simulink model "soc_estimation"  (R2024b)
settings: Solver=FixedStepAuto  StartTime=0.0  StopTime=6*3600  RelTol=1e-3
undefined symbols (not defined in the file): R, Ts
libraries: BatteryEstimators x8, simulink x4, nesl_utility x4, fl_lib x3, batteryecm_lib x1
settings Model: Creator=andri  LastModifiedBy=andri
settings OptimizationCC: DefaultParameterBehavior=Inlined  UseDivisionForNetSlopeComputation=on  GainParamInheritBuiltInType=on  UseFloatMulNetSlope=on  InlineInvariantSignals=on  EnhancedBackFolding=on  PassReuseOutputArgsAs=Individual arguments  ZeroExternalMemoryAtStartup=off  ZeroInternalMemoryAtStartup=off  EfficientFloat2IntCast=on  OptimizeBlockOrder=speed  DifferentSizesBufferReuse=on  OptimizationCustomize=off  EfficientTunableParamExpr=on
settings DebuggingCC: ParameterTunabilityLossMsg=error  SFUnexpectedBacktrackingDiag=warning  SFNoUnconditionalDefaultTransitionDiag=warning
settings HardwareCC: TargetBitPerLong=64  TargetBitPerPointer=64  TargetBitPerSizeT=64  TargetBitPerPtrDiffT=64  TargetLongLongMode=on  TargetIntDivRoundTo=Zero  TargetEndianess=LittleEndian  TargetWordSize=64  TargetHWDeviceType=MATLAB Host  ProdEqTarget=off
settings SFSimCC: MATLABDynamicMemAlloc=off  SimTargetLang=C++
settings RTWCC: Description=AUTOSAR  SystemTargetFile=autosar.tlc  GenCodeOnly=on  TemplateMakefile=ert_default_tmf  GenerateReport=on  BuildConfiguration=Debug  LaunchReport=on  DataTypeReplacement=CDataTypesFixedWidth
settings CodeAppCC: ForceParamTrailComments=on  IgnoreCustomStorageClasses=off  OperatorAnnotations=on  SimulinkDataObjDesc=on  SFDataObjDesc=on  InsertBlockDesc=on  EnableCustomComments=on
settings STFCustomTargetCC: TargetLangStandard=C99 (ISO)  MultiwordLength=256  ParMdlRefBuildCompliant=on  CompOptLevelCompliant=on  IncludeMdlTerminateFcn=off  CombineOutputUpdateFcns=on  SuppressErrorStatus=on  ERTCustomFileBanners=on  SupportNonFinite=off  SupportComplex=off  SupportContinuousTime=off  SupportNonInlinedSFcns=off  RemoveResetFunc=on  MATLABClassNameForMDSCustomization=Simulink.SoftwareTarget.ERTCustomization  AutosarCompliant=on  UseToolchainInfoCompliant=on  LookupTableObjectStructAxisOrder=2,1,3,4,...  LUTObjectStructOrderEvenSpacing=Size,Table,Breakpoints  SystemTargetFile=autosar.tlc
settings ERTTargetCC: TargetLangStandard=C99 (ISO)  ConcurrentExecutionCompliant=off  IncludeMdlTerminateFcn=off  SuppressErrorStatus=on  SupportNonFinite=off  SupportComplex=off  ModelStepFunctionPrototypeControlCompliant=off  CPPClassGenCompliant=off  AutosarCompliant=on  LookupTableObjectStructAxisOrder=2,1,3,4,...  LUTObjectStructOrderEvenSpacing=Size,Table,Breakpoints  ERTCustomFileTemplate=example_file_process.tlc  BooleanTrueId=TRUE  BooleanFalseId=FALSE

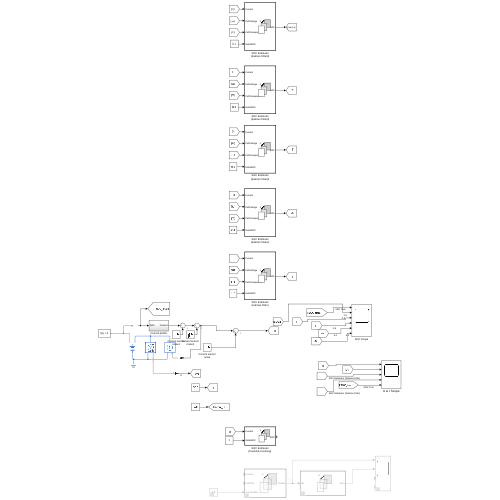
[thumbnail: Simulink's stored preview of the top-level diagram]
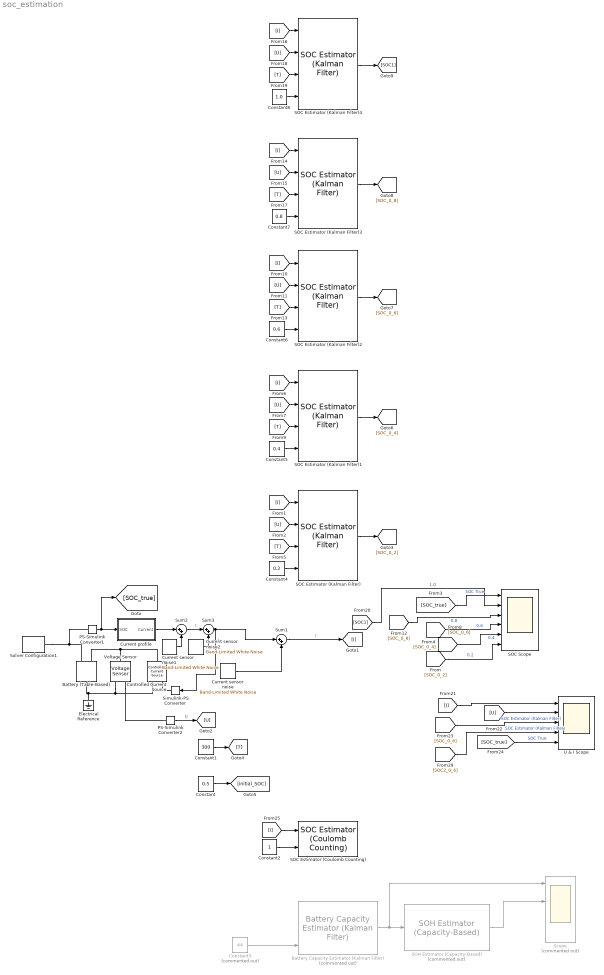
== system soc_estimation ==
  Battery (Table-Based) : batteryecm_lib/Battery (Table-Based)  SOC_vec=SOC  T_dependence=simscape.enum.tablebattery.temperature_dependence.yes  prm_dir=simscape.enum.tablebattery.prm_dir.noCurrentDirectionality  T_vec=T K  V0_mat=Em V  V0_vec=[3.5057, 3.566, 3.6337, 3.7127, 3.9259, 4.0777, 4.1928] V  V_range=[0, inf] V  R0_mat=R0 Ohm  R0_vec=[.0085, .0085, .0087, .0082, .0083, .0085, .0085] Ohm  R0_dis_mat=[.0117, .0085, .009; .011, .0085, .009; .0114, .0087, .0092; .0107, .0082, .0088; .0107, .0083, .0091; .0113, .0085, .0089; .0116, .0085, .0089] Ohm  R0_dis_vec=[.0085, .0085, .0087, .0082, .0083, .0085, .0085] Ohm  R0_ch_mat=[.0117, .0085, .009; .011, .0085, .009; .0114, .0087, .0092; .0107, .0082, .0088; .0107, .0083, .0091; .0113, .0085, .0089; .0116, .0085, .0089] Ohm  R0_ch_vec=[.0085, .0085, .0087, .0082, .0083, .0085, .0085] Ohm  AH=44 A*hr  prm_leak=simscape.enum.tablebattery.prm_leak.disabled  Rleak_vec=[8000, 7000, 6000] Ohm  Rleak=7e3 Ohm  extrapolation_option=simscape.enum.extrapolation.linear  SOC_port=simscape.enum.tablebattery.enable.yes  prm_dyn=simscape.enum.tablebattery.prm_dyn.rc2  R1_mat=R1 Ohm  R1_vec=[.0029, .0024, .0026, .0016, .0023, .0018, .0017] Ohm  tau1_mat=T1 s  tau1_vec=[36, 45, 105, 29, 77, 33, 39] s  R2_mat=R2 Ohm  R2_vec=[.0029, .0024, .0026, .0016, .0023, .0018, .0017] Ohm  tau2_mat=T2 s  tau2_vec=[36, 45, 105, 29, 77, 33, 39] s  R3_mat=[.0109, .0029, .0013; .0069, .0024, .0012; .0047, .0026, .0013; .0034, .0016, .001; .0033, .0023, .0014; .0033, .0018, .0011; .0028, .0017, .0011] Ohm  R3_vec=[.0029, .0024, .0026, .0016, .0023, .0018, .0017] Ohm  tau3_mat=[20, 36, 39; 31, 45, 39; 109, 105, 61; 36, 29, 26; 59, 77, 67; 40, 33, 29; 25, 39, 33] s  tau3_vec=[36, 45, 105, 29, 77, 33, 39] s  R4_mat=[.0109, .0029, .0013; .0069, .0024, .0012; .0047, .0026, .0013; .0034, .0016, .001; .0033, .0023, .0014; .0033, .0018, .0011; .0028, .0017, .0011] Ohm  R4_vec=[.0029, .0024, .0026, .0016, .0023, .0018, .0017] Ohm  tau4_mat=[20, 36, 39; 31, 45, 39; 109, 105, 61; 36, 29, 26; 59, 77, 67; 40, 33, 29; 25, 39, 33] s  tau4_vec=[36, 45, 105, 29, 77, 33, 39] s  R5_mat=[.0109, .0029, .0013; .0069, .0024, .0012; .0047, .0026, .0013; .0034, .0016, .001; .0033, .0023, .0014; .0033, .0018, .0011; .0028, .0017, .0011] Ohm  R5_vec=[.0029, .0024, .0026, .0016, .0023, .0018, .0017] Ohm  tau5_mat=[20, 36, 39; 31, 45, 39; 109, 105, 61; 36, 29, 26; 59, 77, 67; 40, 33, 29; 25, 39, 33] s  tau5_vec=[36, 45, 105, 29, 77, 33, 39] s  prm_fade=simscape.enum.tablebattery.prm_fade.tableN  N0=100  dV0=0  dR0=0  dAH=0  dRleak=0  dR1=0  dR2=0  dR3=0  dR4=0  dR5=0  N0vec=[1,5,10,20,30]  Tfadevec=[298.15, 323.15] K  dV0vec=[0, 0, 0, 0, 0]  dR0vec=[0, 0, 0, 0, 0]  dAHvec=[-1.0, 2.5, -5.0, -7.5, -10.0]  dRleakvec=[0, 0, 0, 0]  dR1vec=[0, 0, 0, 0, 0]  dR2vec=[0, 0, 0, 0, 0]  dR3vec=[0, 0, 0, 0]  dR4vec=[0, 0, 0, 0]  dR5vec=[0, 0, 0, 0]  dV0mat=[0, 0; 0, 0; 0, 0; 0, 0]  dR0mat=[0, 0; 0, 0; 0, 0; 0, 0]  dAHmat=[0, 0; 0, 0; 0, 0; 0, 0]  dRleakmat=[0, 0; 0, 0; 0, 0; 0, 0]  dR1mat=[0, 0; 0, 0; 0, 0; 0, 0]  dR2mat=[0, 0; 0, 0; 0, 0; 0, 0]  dR3mat=[0, 0; 0, 0; 0, 0; 0, 0]  dR4mat=[0, 0; 0, 0; 0, 0; 0, 0]  dR5mat=[0, 0; 0, 0; 0, 0; 0, 0]  prm_age_modeling=simscape.enum.tablebattery.prm_age_modeling.equation  storage_dt_age_vec=[0] d  storage_T_age_vec=[273] K  prm_age_OCV=simscape.enum.tablebattery.prm_age_OCV.OCV  OCV_age=0.9  SOC_age=0.6  prm_age_resistance=simscape.enum.tablebattery.prm_age.disabled  OCV_scaling_age_resistance=2.2134e6  OCV_offset_age_resistance=1.632e6  temp_exp_age_resistance=0.515833569 V  t_exp_age_resistance=0.75  T_age_vec_resistance=[273.15, 298.15, 323.15] K  dt_age_vec_resistance=[0, 90, 180, 270] d  dR0_age_vec=[0, 0, 0]  t_meas_dR0_age=100 d  dR0_age_mat=[0, 0, 0; 0, 0, 0; 0, 0, 0; 0, 0, 0]  prm_age_capacity=simscape.enum.tablebattery.prm_age.disabled  OCV_scaling_age_capacity=1.5097e07  OCV_offset_age_capacity=8.3625e06  temp_exp_age_capacity=0.6011 V  t_exp_age_capacity=0.75  T_age_vec_capacity=[273.15, 298.15, 323.15] K  dt_age_vec_capacity=[0, 90, 180, 270] d  dAH_age_vec=[0, 0, 0]  t_meas_dAH_age=100 d  dAH_age_mat=[0, 0, 0; 0, 0, 0; 0, 0, 0; 0, 0, 0]  thermal_port=simscape.enum.thermaleffects.omit  temperature=298.15 K  thermal_mass=100 J/K  i_specify=off  i_priority=None  i=0 A  i_nominal_specify=off  i_nominal_value=1  i_nominal_unit=A  v_specify=off  v_priority=None  v=0 V  v_nominal_specify=off  v_nominal_value=1  v_nominal_unit=V  stateOfCharge_specify=off  stateOfCharge_priority=High  stateOfCharge=1  stateOfCharge_nominal_specify=off  stateOfCharge_nominal_value=1  stateOfCharge_nominal_unit=1  num_cycles_specify=off  num_cycles_priority=High  num_cycles=0  num_cycles_nominal_specify=off  num_cycles_nominal_value=1  num_cycles_nominal_unit=1  cell_temperature_specify=off  cell_temperature_priority=High  cell_temperature=298.15 K  cell_temperature_nominal_specify=off  cell_temperature_nominal_value=1  cell_temperature_nominal_unit=K
      settings: InternalSimscapePortConfiguration="{\"Bottom\":[],\"Left\":[{\"id\":\"p\",\"label\":\"+\",\"type\":\"foundation.electrical.electrical\"},{\"id\":\"soc\",\"label\":\"SOC\",\"type\":\"output\"}],\"Right\":[{\"id\":\"n\",\"label\":\"-\",\"type\":\"foundation.electrical.electrical\"}],\"Top\":[]}"
      settings: LibrarySourceBlock=|
      | batt_lib/Cells/Battery
      | (Table-Based)
  Battery Capacity Estimator (Kalman Filter) : BatteryEstimators/Battery Capacity Estimator (Kalman Filter)  Commented=on  CurrentInputPartition=off  filterType=Extended Kalman filter  alpha=1  beta=2  kappa=0  Q=3e-4  R=5e-7  P0=1e-8  Ts=1
      settings: LibrarySourceBlock=|
      | batt_sl_lib/Estimators/Battery Capacity Estimator
      | (Kalman Filter)
  Constant : Constant  Value=0.5
  Constant1 : Constant  Value=300
  Constant2 : Constant
  Constant3 : Constant  Commented=on  Value=44
  Constant4 : Constant  Value=0.2
  Constant5 : Constant  Value=0.4
  Constant6 : Constant  Value=0.6
  Constant7 : Constant  Value=0.8
  Constant8 : Constant  Value=1.0
  Controlled Current Source : fl_lib/Electrical/Electrical Sources/Controlled Current Source
  Current profile : Subsystem
  Current sensor noise : simulink/Sources/Band-Limited White Noise  Cov=1e-4  Ts=0.1  seed=1234
  Current sensor noise1 : simulink/Sources/Band-Limited White Noise  Cov=0.005  Ts=0.1  seed=1234
  Current sensor noise2 : simulink/Sources/Band-Limited White Noise  Cov=0.01  Ts=1  seed=1234
  Electrical Reference : fl_lib/Electrical/Electrical Elements/Electrical Reference
  PS-Simulink Converter1 : nesl_utility/PS-Simulink Converter  PhysicalDomain=network_engine_domain  SubClassName=ps_output  LeftPortType=input  RightPortType=output  PseudoPeriodic=off  Frequencies=[]  VectorFormat=inherit  Unit=inherit  AffineConversion=off
  PS-Simulink Converter2 : nesl_utility/PS-Simulink Converter  PhysicalDomain=network_engine_domain  SubClassName=ps_output  LeftPortType=input  RightPortType=output  PseudoPeriodic=off  Frequencies=[]  VectorFormat=inherit  Unit=inherit  AffineConversion=off
  "SOC Estimator (Coulomb Counting) " : BatteryEstimators/SOC Estimator (Coulomb Counting)  CurrentInputPartition=on  AH=80  Ts=1
      settings: LibrarySourceBlock=|
      | batt_sl_lib/Estimators/SOC Estimator
      | (Coulomb Counting)
  SOC Estimator (Kalman Filter){,1..4} (5 alike) : BatteryEstimators/SOC Estimator (Kalman Filter)  CurrentInputPartition=off  filterType=Extended Kalman filter  alpha=1  beta=2  kappa=0  Q=Q  Q_2RC=Q  R=R  P0=P  P0_2RC=P  Ts=1  chargeDynamics=Two time-constant dynamics  SOC_vec=SOC  T_vec=T  R0_mat=R0  R1_mat=R1  tau1_mat=T1  R2_mat=R2  tau2_mat=T2  V0_mat=Em  AH=44
  SOC Scope : Scope  NumInputPorts=6
  SOH Estimator (Capacity-Based) : BatteryEstimators/SOH Estimator (Capacity-Based)  Commented=on  AH_new=44  AH_eol=34
      settings: LibrarySourceBlock=batt_sl_lib/Estimators/SOH Estimator (Capacity-Based)
  Scope : Scope  Commented=on  NumInputPorts=4
  Simulink-PS Converter : nesl_utility/Simulink-PS Converter  PhysicalDomain=network_engine_domain  SubClassName=ps_input  LeftPortType=input  RightPortType=output  PseudoPeriodic=off  Frequencies=[]  NoiseDistribution=none  NoiseParameters=[]  Unit=1  AffineConversion=off  FilteringAndDerivatives=provide  SimscapeFilterOrder=1  InputFilterTimeConstant=0.001  UdotUserProvided=0
  Solver Configuration1 : nesl_utility/Solver Configuration  PhysicalDomain=network_engine_domain  SubClassName=solver  LeftPortType=input  RightPortType=generic  Tones=[]  Harmonics=[]  SimulateNoise=off  Profile=off  UseLocalSampling=off  EnableSwitchedLinearOptims=on  FrequencyDomain=off  UseCCode=off  RelTol=0.001  AbsTol=0.001  MinStep=1e-09  ToWorkspace=off  RevertToSquareIcSolve=off  NumHomotopyIterations=100  PhasorMode=off  PhasorModeNumHarmonics=1  ConsistencySolver=NEWTON_XTOL_AFTER_FTOL  IndexReductionMethod=DerivativeReplacement  DoDC=off  ResidualTolerance=1e-09  ConsistencyTolSource=GLOBAL  ConsistencyAbsTol=0.001  ConsistencyRelTol=0.001  ConsistencyTolFactor=0.001  UseLocalSolver=on  LocalSolverChoice=NE_BACKWARD_EULER_ADVANCER  ResolveIndetEquations=on  FunctionEvalNumThread=1  LocalSolverSampleTime=1  DoFixedCost=on  MaxNonlinIter=3  MaxModeIter=2  ComputeImpulses=off  ImpulseIterations=2  LinearAlgebra=auto  LinearAlgebraNumThread=0  EquationFormulation=NE_TIME_EF  DelaysMemoryBudget=1024  AutomaticFiltering=on  FilteringTimeConstant=0.001  PartitionStorageMethod=AS_NEEDED  PartitionMemoryBudget=1024  PartitionMethod=ROBUST  MultibodyUseLocalSolver=off  MultibodyLocalSolverChoice=ODE1  MultibodyLocalSolverSampleTime=0.001
  Sum1 : Sum  Inputs=|++
  Sum2 : Sum  Inputs=|++
  Sum3 : Sum  Inputs=|++
  U & I Scope : Scope  NumInputPorts=5
  Voltage Sensor : fl_lib/Electrical/Electrical Sensors/Voltage Sensor
  wires:
  Current sensor noise/1 -> Sum1/2
  Constant2/1 -> "SOC Estimator (Coulomb Counting) "/2
  SOH Estimator (Capacity-Based)/1 -> Scope/2
  Battery Capacity Estimator (Kalman Filter)/1 -> SOH Estimator (Capacity-Based)/1, Scope/1
  Constant3/1 -> Battery Capacity Estimator (Kalman Filter)/3
  PS-Simulink Converter1/1 -> Current profile/1(SOC), [SOC_true]
  Constant1/1 -> [T]
  SOC Estimator (Kalman Filter)/1 -> [SOC_0_2]
  Constant/1 -> [initial_SOC]
  [I] -> SOC Estimator (Kalman Filter)/1
  [U] -> SOC Estimator (Kalman Filter)/2
  [T] -> SOC Estimator (Kalman Filter)/3
  Constant4/1 -> SOC Estimator (Kalman Filter)/4
  SOC Estimator (Kalman Filter)1/1 -> [SOC_0_4]
  Constant5/1 -> SOC Estimator (Kalman Filter)1/4
  [U] -> SOC Estimator (Kalman Filter)1/2
  [I] -> SOC Estimator (Kalman Filter)1/1
  [T] -> SOC Estimator (Kalman Filter)1/3
  SOC Estimator (Kalman Filter)2/1 -> [SOC_0_6]
  [U] -> SOC Estimator (Kalman Filter)2/2
  [I] -> SOC Estimator (Kalman Filter)2/1
  [T] -> SOC Estimator (Kalman Filter)2/3
  SOC Estimator (Kalman Filter)3/1 -> [SOC_0_8]
  Constant7/1 -> SOC Estimator (Kalman Filter)3/4
  [U] -> SOC Estimator (Kalman Filter)3/2
  [I] -> SOC Estimator (Kalman Filter)3/1
  [T] -> SOC Estimator (Kalman Filter)3/3
  Constant6/1 -> SOC Estimator (Kalman Filter)2/4
  [SOC_true] -> SOC Scope/1  "SOC True"
  [SOC_0_6] -> SOC Scope/4  "0.6"
  [SOC_0_8] -> SOC Scope/3  "0.8"
  [SOC_0_4] -> SOC Scope/5  "0.4"
  [SOC_0_2] -> SOC Scope/6  "0.2"
  [I] -> SOC Estimator (Kalman Filter)4/1
  [U] -> SOC Estimator (Kalman Filter)4/2
  SOC Estimator (Kalman Filter)4/1 -> [SOC1]
  [T] -> SOC Estimator (Kalman Filter)4/3
  Constant8/1 -> SOC Estimator (Kalman Filter)4/4
  [SOC1] -> SOC Scope/2  "1.0"
  [SOC_true] -> U & I Scope/5  "SOC True"
  [I] -> "SOC Estimator (Coulomb Counting) "/1
  [I] -> U & I Scope/1
  [U] -> U & I Scope/2
  [SOC_0_6] -> U & I Scope/3  "SOC Estimator (Kalman Filter)"
  [SOC2_0_6] -> U & I Scope/4  "SOC Estimator (Kalman Filter)"
  Sum1/1 -> [I]  "I"
  Current profile/1(Current) -> Sum2/1
  Current sensor noise1/1 -> Sum2/2
  Current sensor noise2/1 -> Sum3/2
  Sum2/1 -> Sum3/1  "I"
  Sum3/1 -> Simulink-PS Converter/1, Sum1/1  "I"
  PS-Simulink Converter2/1 -> [U]  "U"
  connections:
  Voltage Sensor/RConn2 -- Battery (Table-Based)/RConn1 -- Electrical Reference/LConn1 -- Controlled Current Source/RConn2
  Voltage Sensor/LConn1 -- Controlled Current Source/LConn1 -- Battery (Table-Based)/LConn1
  Voltage Sensor/RConn1 -- PS-Simulink Converter2/LConn1
  Simulink-PS Converter/RConn1 -- Controlled Current Source/RConn1
  Battery (Table-Based)/LConn2 -- Solver Configuration1/RConn1 -- PS-Simulink Converter1/LConn1

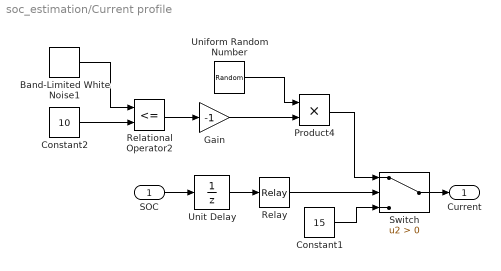
== system soc_estimation/Current profile ==
  SOC : Inport
  Band-Limited White Noise1 : simulink/Sources/Band-Limited White Noise  Cov=1  Ts=50  seed=[23341]
  Constant1 : Constant  Value=15
  Constant2 : Constant  Value=10
  Gain : Gain  Gain=-1
  Product4 : Product
  Relational Operator2 : RelationalOperator  Operator=<=  OutDataTypeStr=boolean  RndMeth=Simplest  InputSameDT=off
  Relay : Relay  OnSwitchValue=0.9  OffSwitchValue=0.3  OffOutputValue=-1
  Switch : Switch  Criteria=u2 > Threshold  SaturateOnIntegerOverflow=off  InputSameDT=off
  Uniform Random Number : UniformRandomNumber  Minimum=4  Maximum=7  SampleTime=600
  Unit Delay : UnitDelay  SampleTime=Ts  HasFrameUpgradeWarning=on
  Current : Outport
  wires:
  SOC/1 -> Unit Delay/1
  Constant1/1 -> Switch/3
  Relay/1 -> Switch/2
  Product4/1 -> Switch/1
  Unit Delay/1 -> Relay/1
  Switch/1 -> Current/1
  Uniform Random Number/1 -> Product4/1
  Band-Limited White Noise1/1 -> Relational Operator2/1
  Gain/1 -> Product4/2
  Relational Operator2/1 -> Gain/1
  Constant2/1 -> Relational Operator2/2
